simulink model "pid"  (Simulink 9.0)
settings: Solver=ode23  StartTime=0.0  StopTime=50  MaxStep=10  RelTol=1e-3  AbsTol=1e-3  EnableMultiTasking=on
undefined symbols (not defined in the file or in its folder): D, den, I, K, num, sfunyst, T
settings Model: Creator=Marco Campi  LastModifiedBy=algoc  ExtModeTrigMode=oneshot  ExtModeArmWhenConnect=off
settings DataIOCC: SignalLoggingSaveFormat=ModelDataLogs  SaveOutput=off  SaveTime=off
settings OptimizationCC: BlockReduction=off  BooleanDataType=off  ExpressionDepthLimit=2147483647  InitFltsAndDblsToZero=on
settings DebuggingCC: SaveWithParameterizedLinksMsg=none  SignalResolutionControl=TryResolveAllWithWarning  MultiTaskDSMMsg=warning  MultiTaskCondExecSysMsg=none  FcnCallInpInsideContextMsg=warning  StateNameClashWarn=warning  StrictBusMsg=None
settings HardwareCC: TargetUnknown=on
settings GRTTargetCC: TargetFcnLib=ansi_tfl_tmw.mat  CombineOutputUpdateFcns=off  GRTInterface=on

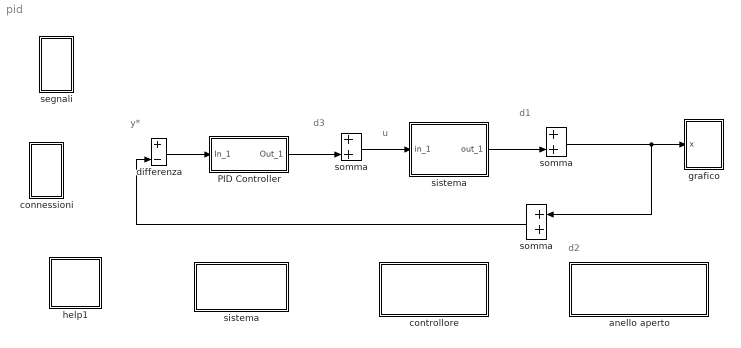
== system pid ==
  note: y*
  note: d3
  note: u
  note: d1
  note: d2
  " somma " : Sum  SaturateOnIntegerOverflow=on  InputSameDT=on  OutDataTypeStr=Inherit: Same as first input
  PID Controller : Subsystem
      settings: OpenFcn=blocca
      mask Help: This block implements a PID controller where parameters are entered for the Proportional, Integral and Derivative terms. Unmask this block to see how it works. The derivative term is implemented using a true derivative block.
      mask Display: disp('PID')
  anello aperto : Subsystem
      mask Display: disp('analisi\n in anello aperto')
  connessioni : Subsystem
  controllore : Subsystem
      mask Display: disp('PID')
  differenza : Sum  Inputs=+-  SaturateOnIntegerOverflow=on  InputSameDT=on  OutDataTypeStr=Inherit: Same as first input
  grafico : Subsystem  mask(Storage scope.){MaskParam1=10, MaskParam2=-10, MaskParam3=10, npts=2000, color='b-/r-/g--/c-./w:/m*/ro/b+'}
      mask prompts: MaskParam1 "Initial Time Range:"; MaskParam2 "Initial y-min:"; MaskParam3 "Initial y-max:"; npts "Storage pts.:"; color "Line type (rgbw-.:xo):"
      mask help:
      | Storage scope using MATLAB graph window.
      | Enter plotting ranges and line type.
      mask init:
      | ax = [0, MaskParam1, MaskParam2, MaskParam3]; dt=-1;
      mask Help: This block uses a MATLAB figure window to plot the input signal.  The graph limits are automatically scaled to the min and max values of the signal stored in the scope's signal buffer.  Line type must be in quotes.  See the M-file sfunyst.m.
      mask Display: plot(0,0,100,100,[83,76,63,52,42,38,28,16,11,84,11,11,11,90,90,11],[75,58,47,54,72,80,84,74,65,65,65,90,40,40,90,90])
  help1 : Subsystem
      mask Display: disp('?')
  segnali : Subsystem
  sistema : Subsystem
      mask Display: disp('sistema')
  "sistema " : Subsystem
      settings: OpenFcn=blocca
      mask Display: disp('sistema')
  somma : Sum  SaturateOnIntegerOverflow=on  InputSameDT=on  OutDataTypeStr=Inherit: Same as first input
  "somma " : Sum  SaturateOnIntegerOverflow=on  InputSameDT=on  OutDataTypeStr=Inherit: Same as first input
  wires:
  "sistema "/1(out_1) -> "somma "/2
  " somma "/1 -> differenza/2
  differenza/1 -> PID Controller/1(In_1)
  "somma "/1 -> " somma "/1, grafico/1(x)
  PID Controller/1(Out_1) -> somma/2
  somma/1 -> "sistema "/1(in_1)

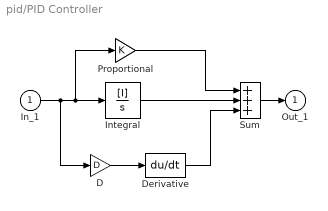
== system pid/PID Controller ==
  In_1 : Inport
  D : Gain  Gain=D  SaturateOnIntegerOverflow=on  OutDataTypeStr=Inherit: Same as input  ParamDataTypeStr=Inherit: Same as input
  Derivative : Derivative
  Integral : TransferFcn  Numerator=[I]  Denominator=[1 0]
  Proportional : Gain  Gain=K  SaturateOnIntegerOverflow=on  OutDataTypeStr=Inherit: Same as input  ParamDataTypeStr=Inherit: Same as input
  Sum : Sum  Inputs=+++  SaturateOnIntegerOverflow=on  InputSameDT=on  OutDataTypeStr=Inherit: Same as first input
  Out_1 : Outport
  wires:
  D/1 -> Derivative/1
  Sum/1 -> Out_1/1
  In_1/1 -> D/1, Integral/1, Proportional/1
  Derivative/1 -> Sum/3
  Integral/1 -> Sum/2
  Proportional/1 -> Sum/1

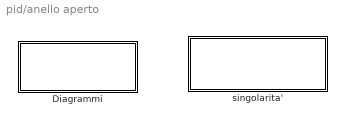
== system pid/anello aperto ==
  Diagrammi : Subsystem
      mask Display: disp('diagrammi\n  \n (Bode e Nyquist)')
  singolarita' : Subsystem  mask(singolarita' della f.d.t.){}
      settings: OpenFcn=sing_tot
      mask Display: disp('singolarità,\n guadagno e ritardo')

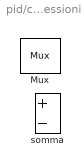
== system pid/connessioni ==
  Mux : Mux  Inputs=2
  somma : Sum  Inputs=+-  SaturateOnIntegerOverflow=on  InputSameDT=on  OutDataTypeStr=Inherit: Same as first input

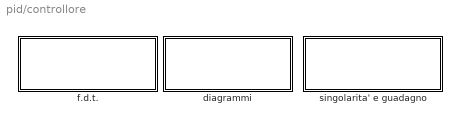
== system pid/controllore ==
  diagrammi : Subsystem
      mask Display: disp('diagramma di Bode')
  f.d.t. : Subsystem  mask(assegnamento controllore){}
      settings: OpenFcn=ass2_cn
      mask Display: disp('inserimento f.d.t.')
  singolarita' e guadagno : Subsystem  mask(singolarita' della f.d.t.){}
      settings: OpenFcn=sing_c
      mask Display: disp('singolarità e guadagno')

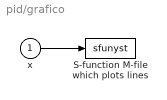
== system pid/grafico ==
  x : Inport
  "S-function M-file which plots lines " : S-Function  LoadFcn=sfunyst([],[],[],'LoadBlock')  FunctionName=sfunyst  Parameters=ax, color, npts, dt  SFunctionDeploymentMode=off  EnableBusSupport=off
      settings: CopyFcn=sfunyst([],[],[],'CopyBlock')  DeleteFcn=sfunyst([],[],[],'DeleteBlock')
  wires:
  x/1 -> "S-function M-file which plots lines "/1

== system pid/help1 ==
  note: i blocchi con l'ombreggiatura consentono
  note: - l'inserimento della funzione di trasferimento
  note: - l'ottenimento dei diagrammi di Bode e di Nyquist
  note: - la determinazione delle singolarità, del guadagno e del ritardo

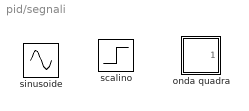
== system pid/segnali ==
  onda quadra : Subsystem  mask(Pulse Generator){Ts=2, du=1, ht=1, stt=0}
      mask prompts: Ts "Pulse period (secs):"; du "Pulse width:"; ht "Pulse height:"; stt "Pulse start time:"
      mask help: Pulse Generator.
      mask init:
      | ini=ones(length(ht),1); st1=rem(stt,Ts); st2=rem(stt+du,Ts);if(Ts<=1.2*du),ini=zeros(length(ht),1);end;
      mask Help: Pulse generator which ensures pulse\ntransitions are hit. Provides a vector of pulses when the height is entered as a vector.\nUnmask to see how it works.
      mask Display: plot(0,0,100,100,[90,75,75,60,60,35,35,20,20,10],[20,20,80,80,20,20,80,80,20,20])
  scalino : Step  Time=0
  sinusoide : Sin

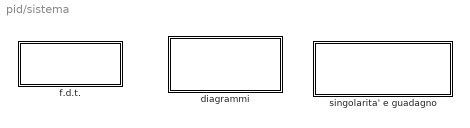
== system pid/sistema ==
  diagrammi : Subsystem
      mask Display: disp('diagrammi\n  \n (Bode e Nyquist)')
  f.d.t. : Subsystem  mask(assegnamento sistema){}
      settings: OpenFcn=ass_sis
      mask Display: disp('inserimento\n f.d.t.')
  singolarita' e guadagno : Subsystem  mask(singolarita' della f.d.t.){}
      settings: OpenFcn=sing_s
      mask Display: disp('singolarità,\n guadagno e ritardo')

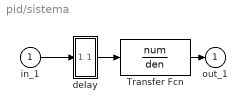
== system pid/sistema  ==
  in_1 : Inport
  Transfer Fcn : TransferFcn  Numerator=num  Denominator=den
  delay : Subsystem
  out_1 : Outport
  wires:
  Transfer Fcn/1 -> out_1/1
  delay/1(out_1) -> Transfer Fcn/1
  in_1/1 -> delay/1(in_1)

== system pid/anello aperto/Diagrammi ==
  Bode : Subsystem
      settings: OpenFcn=bode_tot
      mask Display: disp('Bode')
  Nyquist : Subsystem
      settings: OpenFcn=nyq_tot
      mask Display: disp('Nyquist')

== system pid/anello aperto/singolarita' ==
  note: assegna

== system pid/controllore/diagrammi ==
  Bode : Subsystem
      settings: OpenFcn=bode_c
      mask Display: disp('Bode')

== system pid/controllore/f.d.t. ==
  note: assegna

== system pid/controllore/singolarita' e guadagno ==
  note: assegna

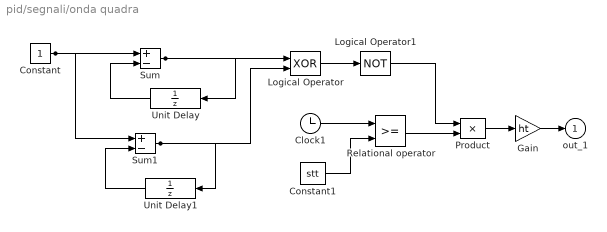
== system pid/segnali/onda quadra ==
  Clock1 : Clock
  Constant : Constant
  Constant1 : Constant  Value=stt
  Gain : Gain  Gain=ht  SaturateOnIntegerOverflow=on  OutDataTypeStr=Inherit: Same as input  ParamDataTypeStr=Inherit: Same as input
  Logical Operator : Logic  Operator=XOR
  Logical Operator1 : Logic  Operator=NOT  Inputs=1
  Product : Product  SaturateOnIntegerOverflow=on  RndMeth=Zero  InputSameDT=on  OutDataTypeStr=Inherit: Same as first input
  Relational operator : RelationalOperator  RndMeth=Nearest  InputSameDT=on
  Sum : Sum  Inputs=+-  SaturateOnIntegerOverflow=on  InputSameDT=on  OutDataTypeStr=Inherit: Same as first input
  Sum1 : Sum  Inputs=+-  SaturateOnIntegerOverflow=on  InputSameDT=on  OutDataTypeStr=Inherit: Same as first input
  Unit Delay : UnitDelay  SampleTime=[Ts,st1]
  Unit Delay1 : UnitDelay  InitialCondition=ini  SampleTime=[Ts,st2]
  out_1 : Outport
  wires:
  Logical Operator1/1 -> Product/1
  Logical Operator/1 -> Logical Operator1/1
  Constant1/1 -> Relational operator/2
  Gain/1 -> out_1/1
  Product/1 -> Gain/1
  Relational operator/1 -> Product/2
  Clock1/1 -> Relational operator/1
  Unit Delay/1 -> Sum/2
  Unit Delay1/1 -> Sum1/2
  Constant/1 -> Sum/1, Sum1/1
  Sum/1 -> Unit Delay/1, Logical Operator/1
  Sum1/1 -> Unit Delay1/1, Logical Operator/2

== system pid/sistema/diagrammi ==
  Bode : Subsystem
      settings: OpenFcn=bode_sis
      mask Display: disp('Bode')
  Nyquist : Subsystem
      settings: OpenFcn=nyq_sis
      mask Display: disp('Nyquist')

== system pid/sistema/f.d.t. ==
  note: assegna

== system pid/sistema/singolarita' e guadagno ==
  note: assegna

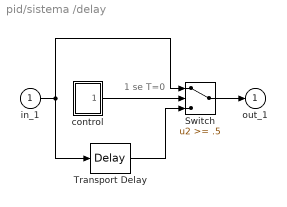
== system pid/sistema /delay ==
  note: 1 se T=0
  in_1 : Inport
  Switch : Switch  Threshold=.5  SaturateOnIntegerOverflow=on  InputSameDT=on
  Transport Delay : TransportDelay  DelayTime=T
  control : Subsystem
  out_1 : Outport
  wires:
  Transport Delay/1 -> Switch/3
  in_1/1 -> Switch/1, Transport Delay/1
  Switch/1 -> out_1/1
  control/1(out_1) -> Switch/2

== system pid/anello aperto/Diagrammi/Bode ==
  note: bode

== system pid/anello aperto/Diagrammi/Nyquist ==
  note: bode

== system pid/controllore/diagrammi/Bode ==
  note: bode

== system pid/sistema/diagrammi/Bode ==
  note: bode

== system pid/sistema/diagrammi/Nyquist ==
  note: bode

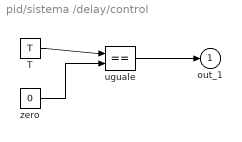
== system pid/sistema /delay/control ==
  T : Constant  Value=T
  uguale : RelationalOperator  Operator===  RndMeth=Nearest  InputSameDT=on
  zero : Constant  Value=0
  out_1 : Outport
  wires:
  zero/1 -> uguale/2
  T/1 -> uguale/1
  uguale/1 -> out_1/1
